simulink model "kinematics"  (R2019a)
settings: Solver=FixedStepAuto  StartTime=0.0  StopTime=10.0  FixedStep=0.01  RelTol=1e-3
settings Model: Creator=chute  LastModifiedBy=chute

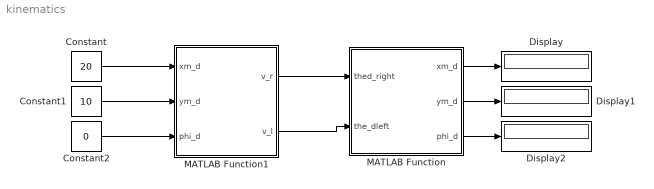
== system kinematics ==
  Constant : Constant  Value=20
  Constant1 : Constant  Value=10
  Constant2 : Constant  Value=0
  Display : Display
  Display1 : Display
  Display2 : Display
  MATLAB Function : MATLAB Function  TreatAsAtomicUnit=on
  MATLAB Function1 : MATLAB Function  TreatAsAtomicUnit=on
  wires:
  MATLAB Function1/1(v_r) -> MATLAB Function/1(thed_right)
  MATLAB Function1/2(v_l) -> MATLAB Function/2(the_dleft)
  Constant/1 -> MATLAB Function1/1(xm_d)
  Constant1/1 -> MATLAB Function1/2(ym_d)
  MATLAB Function/1(xm_d) -> Display/1
  MATLAB Function/2(ym_d) -> Display1/1
  Constant2/1 -> MATLAB Function1/3(phi_d)
  MATLAB Function/3(phi_d) -> Display2/1

== matlab function kinematics/MATLAB Function1 ==
  data: xm_d input; v_r output; v_l output; ym_d input; phi_d input
function [v_r,v_l] = inverse(xm_d,ym_d,phi_d)
W=4;% body
R=5; % Wheel radius
the_d=1/2*()
c1=xm_d/R*
J_t= [cos(phi), sin(phi),W/2;
      [cos(phi), sin(phi)-W/2];
out1 =J_t.*[xm_d;ym_d;phi_d];
v_r=out1(1,1);
v_l=out1(2,1);
end

== matlab function kinematics/MATLAB Function ==
  data: thed_right input; xm_d output; the_dleft input; ym_d output; phi_d output
function [xm_d,ym_d,phi_d] = fcn(thed_right,the_dleft)
W=4;
R =5; % Wheel radius
% right = [R*cos(phi)*the_dot+W*sin(phi)/2;
%        R*sin(phi)*the_dot-W*cos(phi)/2;
%        R];
% % left wheel
% left =[R*cos(phi)*the_dot+W*sin(phi)*phi_dot/2;
%        R*sin(phi)*the_dot-W*cos(phi)*phi_dot/2;
%        R];
 % center
phi=0;
J=[R*cos(phi)/2,R*cos(phi)/2;
    R*sin(phi)/2,R*sin(phi)/2;
    R/W,-R/W];
P_m=J*[thed_right;the_dleft];
xm_d=P_m(1,1);
ym_d=P_m(2,1);
phi_d=P_m(3,1);
